simulink model "close_loop_boost_converter"  (R2018a)
settings: Solver=VariableStepAuto  StartTime=0.0  StopTime=0.2  RelTol=1e-3
libraries: powerlib x11, powerlib_meascontrol x1, simulink x1
settings Model: Creator=asus  LastModifiedBy=asus
settings SolverCC: ZeroCrossAlgorithm=Adaptive
settings DebuggingCC: MaxConsecutiveZCsMsg=none

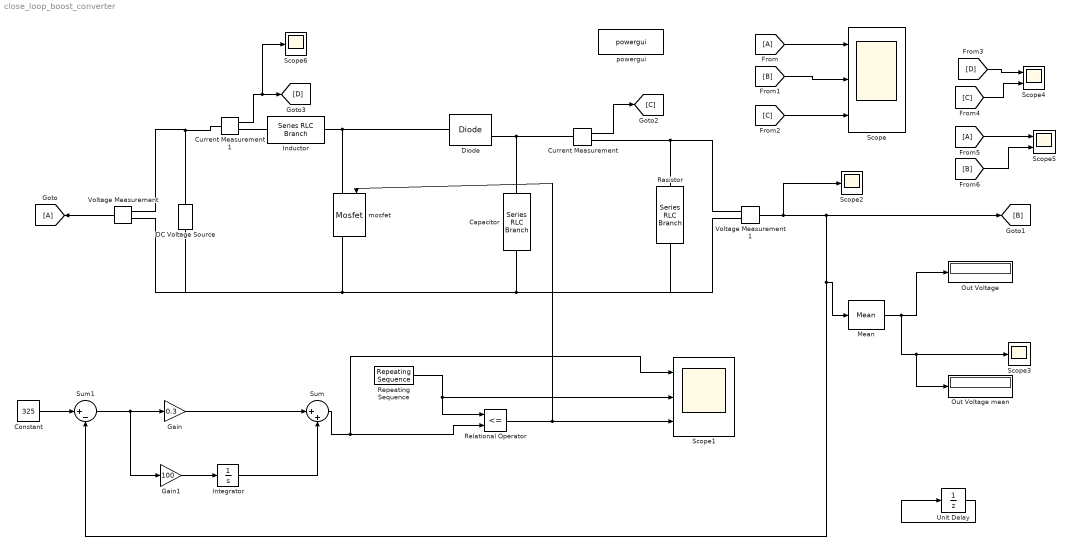
== system close_loop_boost_converter ==
  Capacitor : powerlib/Elements/Series RLC Branch  LConnTagsString=__new0  RConnTagsString=__new0  BranchType=C  Resistance=1  Inductance=1e-3  SetiL0=off  InitialCurrent=0  Capacitance=110e-6  Setx0=off  InitialVoltage=0  Measurements=None
  Constant : Constant  Value=325
  Current Measurement : powerlib/Measurements/Current Measurement  PhasorSimulation=off  OutputType=Complex  PSBequivalent=0
  Current Measurement1 : powerlib/Measurements/Current Measurement  PhasorSimulation=off  OutputType=Complex  PSBequivalent=0
  DC Voltage Source : powerlib/Electrical Sources/DC Voltage Source  Amplitude=183  Measurements=None
  Diode : powerlib/Power Electronics/Diode  Ron=0.001  Lon=0  Vf=0.8  IC=0  UseSnubber=0  Rs=500  Cs=250e-9  Measurements=on
  Gain : Gain  Gain=0.3
  Gain1 : Gain  Gain=100
  Inductor : powerlib/Elements/Series RLC Branch  LConnTagsString=__new0  RConnTagsString=__new0  BranchType=L  Resistance=1  Inductance=1000e-6  SetiL0=off  InitialCurrent=0  Capacitance=1e-6  Setx0=off  InitialVoltage=0  Measurements=None
  Integrator : Integrator
  Mean : powerlib_meascontrol/Measurements/Mean  Freq=60  Vinit=0  Ts=0
  Out Voltage : Display
  Out Voltage mean : Display
  Rasistor : powerlib/Elements/Series RLC Branch  LConnTagsString=__new0  RConnTagsString=__new0  BranchType=R  Resistance=110  Inductance=1e-3  SetiL0=off  InitialCurrent=0  Capacitance=1e-6  Setx0=off  InitialVoltage=0  Measurements=None
  Relational Operator : RelationalOperator  Operator=<=  OutDataTypeStr=boolean  RndMeth=Simplest
  Repeating Sequence : simulink/Sources/Repeating Sequence  rep_seq_t=[0 2.5e-5 5e-5 7.5e-5 1e-4]  rep_seq_y=[0 200 0 -200 0 ]
  Scope : Scope  NumInputPorts=3
  Scope1 : Scope  NumInputPorts=3
  Scope2 : Scope
  Scope3 : Scope
  Scope4 : Scope  NumInputPorts=2
  Scope5 : Scope  NumInputPorts=2
  Scope6 : Scope
  Sum : Sum  Inputs=|++
  Sum1 : Sum  Inputs=|+-
  Unit Delay : UnitDelay  SampleTime=1e-6
  Voltage Measurement : powerlib/Measurements/Voltage Measurement  PhasorSimulation=off  OutputType=Complex  PSBequivalent=0
  Voltage Measurement1 : powerlib/Measurements/Voltage Measurement  PhasorSimulation=off  OutputType=Complex  PSBequivalent=0
  mosfet : powerlib/Power Electronics/Mosfet  Ron=0.1  Lon=0  Rd=0.01  Vfd=0  IC=0  Rs=1e5  Cs=inf  Measurements=on
  powergui : powerlib/powergui  Priority=1  SimulationMode=Continuous  SampleTime=50e-6  frequency=60  Iterations=50  frequencyindice=0  Pbase=100e6  ErrMax=1e-4  UnitsV=kV  UnitsW=MW  buscounter=0  FunctionMessages=off  echomessages=off  EnableUseOfTLC=off  CurrentSourceSwitches=off  DisableSnubberDevices=off  DisableRonSwitches=off  DisableVfSwitches=off  DisplayEquations=off  SolverType=Tustin/Backward Euler (TBE)  Interpol=off  ExternalGateDelay=off  methode=off  Ts=100  x0status=blocks  SPID=on  SwTol=0  HookPort=off  RestoreLinks=warning  ResistiveCurrentMeasurement=off  Frange=[0:2:500]  Ylog=off  Xlog=on  ShowGrid=off  save=off  variable=ZData  structure=0  ZoomFFT=off  StartTime=0.0  cycles=1  DisplayStyle=1  fundamental=60  FreqAxis=off  MaxFrequency=1000  frequencyindicesteady=1  RmsSteady=1  display=off
  wires:
  Current Measurement/1 -> [C]
  [A] -> Scope/1
  [C] -> Scope/3
  [B] -> Scope/2
  Voltage Measurement1/1 -> Scope2/1, [B], Mean/1, Sum1/2
  Repeating Sequence/1 -> Scope1/2, Relational Operator/1
  Relational Operator/1 -> Scope1/3, mosfet/1
  Gain/1 -> Sum/1
  Voltage Measurement/1 -> [A]
  Gain1/1 -> Integrator/1
  Integrator/1 -> Sum/2
  Sum/1 -> Relational Operator/2, Scope1/1
  Constant/1 -> Sum1/1
  Sum1/1 -> Gain1/1, Gain/1
  Unit Delay/1 -> Unit Delay/1
  Mean/1 -> Out Voltage mean/1, Scope3/1, Out Voltage/1
  Current Measurement1/1 -> Scope6/1, [D]
  [D] -> Scope4/1
  [C] -> Scope4/2
  [A] -> Scope5/1
  [B] -> Scope5/2
  connections:
  Inductor/RConn1 -- Diode/LConn1 -- mosfet/LConn1
  Capacitor/RConn1 -- Voltage Measurement1/LConn2 -- Rasistor/RConn1 -- Voltage Measurement/LConn2 -- DC Voltage Source/LConn1 -- mosfet/RConn1
  Capacitor/LConn1 -- Current Measurement/LConn1 -- Diode/RConn1
  Rasistor/LConn1 -- Current Measurement/RConn1 -- Voltage Measurement1/LConn1
  Voltage Measurement/LConn1 -- Current Measurement1/LConn1 -- DC Voltage Source/RConn1
  Current Measurement1/RConn1 -- Inductor/LConn1
